simulink library "droop_lib_new"  (Simulink 8.1)
settings: Solver=ode45  SolverMode=SingleTasking  StartTime=0.0  StopTime=10.0  RelTol=1e-3
values from neighbouring files (symbols this model uses):
  filt = firstOrderDig(50e-3, Tc, 'low')    [Software_BESS_init.m]    (also in firstOrderDig.m = (tau*s) / (tau*s + 1))
  paramDroopFreq2Reac = 0*(1/dPer)    (= 0)    [Software_BESS_init.m]
  paramDroopFreq2Real = 1*(1/dPer)    (= 20)    [Software_BESS_init.m]
  paramDroopVolts2Reac = 1*(1/dPer)    (= 20)    [Software_BESS_init.m]
  paramDroopVolts2Real = 0*(1/dPer)    (= 0)    [Software_BESS_init.m]
  Pgrid = 3e6    (= 3000000)    [Software_BESS_init.m]
  Vgrid = 480/sqrt(3)    [Software_BESS_init.m]
libraries: simulink x1
settings Model: Creator=ch24070  LastModifiedBy=ch24070  CovMetricSettings=dwe  CovHtmlReporting=off  CovSaveCumulativeToWorkspaceVar=off  CovSaveSingleToWorkspaceVar=off  CovExternalEMLEnable=on

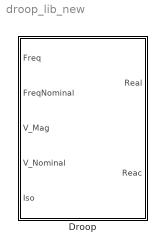
== system droop_lib_new ==
  Droop : Subsystem

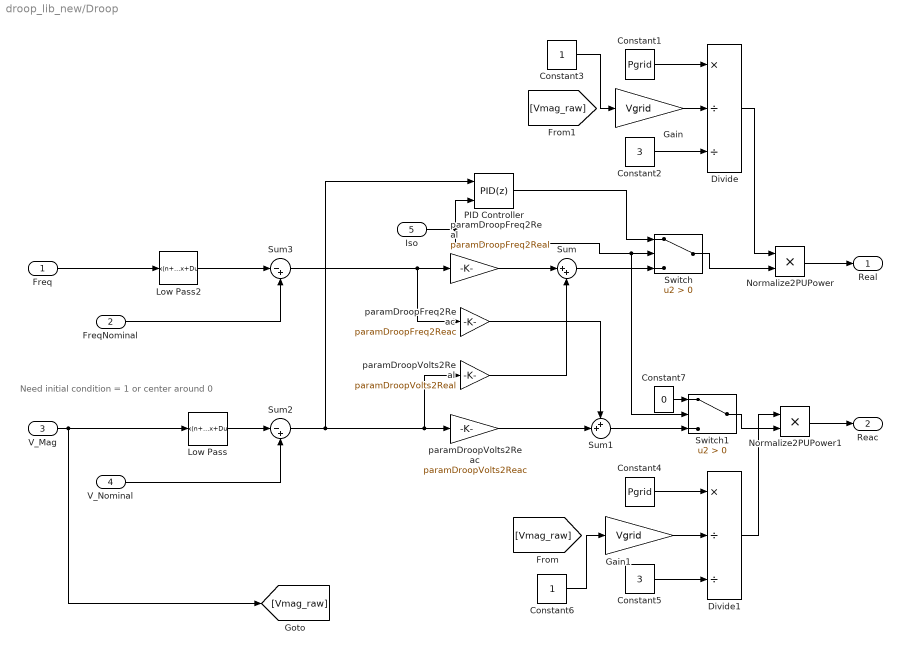
== system droop_lib_new/Droop ==
  note: Need initial condition = 1 or center around 0
  Freq : Inport
  FreqNominal : Inport  Port=2
  V_Mag : Inport  Port=3
  V_Nominal : Inport  Port=4
  Iso : Inport  Port=5
  Constant1 : Constant  Value=Pgrid
  Constant2 : Constant  Value=3
  Constant3 : Constant
  Constant4 : Constant  Value=Pgrid
  Constant5 : Constant  Value=3
  Constant6 : Constant
  Constant7 : Constant  Value=0
  Divide : Product  Inputs=*//
  Divide1 : Product  Inputs=*//
  Gain : Gain  Gain=Vgrid
  Gain1 : Gain  Gain=Vgrid
  Low Pass : DiscreteStateSpace  A=filt.A  B=filt.B  C=filt.C  D=filt.D  X0=1/filt.C  SampleTime=-1
  Low Pass2 : DiscreteStateSpace  A=filt.A  B=filt.B  C=filt.C  D=filt.D  SampleTime=-1
  Normalize2PUPower : Product
  Normalize2PUPower1 : Product
  PID Controller : simulink/Continuous/PID Controller  Controller=PID  TimeDomain=Discrete-time  SampleTime=-1  IntegratorMethod=Forward Euler  FilterMethod=Forward Euler  Form=Parallel  UseFilter=on  ControllerParametersSource=internal  P=10  I=1  D=0  N=100  InitialConditionSource=internal  InitialConditionForIntegrator=0  InitialConditionForFilter=0  ExternalReset=level  LimitOutput=off  UpperSaturationLimit=inf  LowerSaturationLimit=-inf  LinearizeAsGain=on  AntiWindupMode=none  Kb=1  TrackingMode=off  Kt=1  PParamMin=[]  PParamMax=[]  IParamMin=[]  IParamMax=[]  DParamMin=[]  DParamMax=[]  NParamMin=[]  NParamMax=[]  KbParamMin=[]  KbParamMax=[]  KtParamMin=[]  KtParamMax=[]  POutMin=[]  POutMax=[]  IOutMin=[]  IOutMax=[]  DOutMin=[]  DOutMax=[]  NOutMin=[]  NOutMax=[]  KbOutMin=[]  KbOutMax=[]  KtOutMin=[]  KtOutMax=[]  IntegratorOutMin=[]  IntegratorOutMax=[]  FilterOutMin=[]  FilterOutMax=[]  SumOutMin=[]  SumOutMax=[]  SumI1OutMin=[]  SumI1OutMax=[]  SumI2OutMin=[]  SumI2OutMax=[]  SumI3OutMin=[]  SumI3OutMax=[]  SumDOutMin=[]  SumDOutMax=[]  SaturationOutMin=[]  SaturationOutMax=[]  IntegratorContinuousStateAttributes=''  IntegratorStateMustResolveToSignalObject=off  IntegratorRTWStateStorageClass=Auto  FilterContinuousStateAttributes=''  FilterStateMustResolveToSignalObject=off  FilterRTWStateStorageClass=Auto  DifferentiatorICPrevScaledInput=0  DifferentiatorOutMin=[]  DifferentiatorOutMax=[]
  Sum : Sum  Inputs=|++
  Sum1 : Sum  Inputs=++|
  Sum2 : Sum  Inputs=|-+
  Sum3 : Sum  Inputs=|-+
  Switch : Switch  Criteria=u2 > Threshold
  Switch1 : Switch  Criteria=u2 > Threshold
  paramDroopFreq2Reac : Gain  Gain=paramDroopFreq2Reac
  paramDroopFreq2Real : Gain  Gain=paramDroopFreq2Real
  paramDroopVolts2Reac : Gain  Gain=paramDroopVolts2Reac
  paramDroopVolts2Real : Gain  Gain=paramDroopVolts2Real
  Real : Outport
  Reac : Outport  Port=2
  wires:
  Constant7/1 -> Switch1/1
  Sum1/1 -> Switch1/3
  Switch1/1 -> Normalize2PUPower1/2
  Sum2/1 -> paramDroopVolts2Reac/1, paramDroopVolts2Real/1, PID Controller/1
  PID Controller/1 -> Switch/1
  Sum/1 -> Switch/3
  Switch/1 -> Normalize2PUPower/2
  paramDroopFreq2Real/1 -> Sum/1
  Iso/1 -> Switch/2, Switch1/2, PID Controller/2
  Constant3/1 -> Gain/1
  Gain/1 -> Divide/2
  Normalize2PUPower1/1 -> Reac/1
  Normalize2PUPower/1 -> Real/1
  Freq/1 -> Low Pass2/1
  FreqNominal/1 -> Sum3/2
  Low Pass/1 -> Sum2/1
  paramDroopVolts2Real/1 -> Sum/2
  paramDroopFreq2Reac/1 -> Sum1/1
  paramDroopVolts2Reac/1 -> Sum1/2
  Sum3/1 -> paramDroopFreq2Real/1, paramDroopFreq2Reac/1
  V_Nominal/1 -> Sum2/2
  Low Pass2/1 -> Sum3/1
  V_Mag/1 -> Low Pass/1, [Vmag_raw]
  Constant1/1 -> Divide/1
  Constant2/1 -> Divide/3
  Divide/1 -> Normalize2PUPower/1
  Constant4/1 -> Divide1/1
  Constant5/1 -> Divide1/3
  Divide1/1 -> Normalize2PUPower1/1
  Constant6/1 -> Gain1/1
  Gain1/1 -> Divide1/2
